simulink model "Clase03122020_FMyPM"  (R2020b)
settings: Solver=VariableStepAuto  StartTime=0.0  StopTime=10.0  RelTol=1e-3
libraries: commanapbnd3 x3
settings Model: Creator=fer-1  LastModifiedBy=fer-1

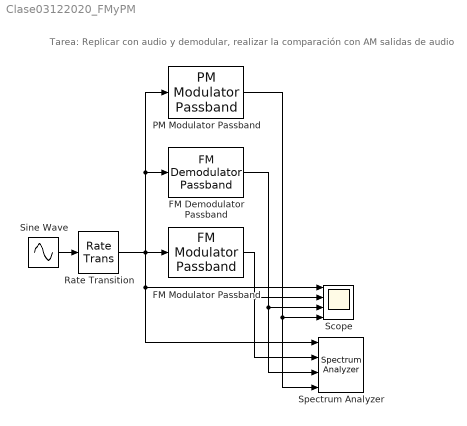
== system Clase03122020_FMyPM ==
  note: Tarea: Replicar con audio y demodular, realizar la comparación con AM salidas de audio
  FM Demodulator Passband : commanapbnd3/FM Demodulator Passband  Fc=300  Ph=0  Kc=50  Ho=100
      settings: SourceProductBaseCode=CM
  FM Modulator Passband : commanapbnd3/FM Modulator Passband  Fc=10e3  Ph=0  Kc=500
      settings: SourceProductBaseCode=CM
  PM Modulator Passband : commanapbnd3/PM Modulator Passband  Fc=1e3  Ph=0  Kc=pi
      settings: SourceProductBaseCode=CM
  Rate Transition : RateTransition  OutPortSampleTime=1/200e3
  Scope : Scope  NumInputPorts=4
  Sine Wave : Sin  Frequency=2*pi*100  SampleTime=0
  Spectrum Analyzer : SpectrumAnalyzer  NumInputPorts=4
  wires:
  FM Modulator Passband/1 -> Spectrum Analyzer/2, Scope/2
  Rate Transition/1 -> PM Modulator Passband/1, FM Demodulator Passband/1, Spectrum Analyzer/1, Scope/1, FM Modulator Passband/1
  Sine Wave/1 -> Rate Transition/1
  FM Demodulator Passband/1 -> Spectrum Analyzer/3, Scope/3
  PM Modulator Passband/1 -> Scope/4, Spectrum Analyzer/4
